simulink model "klademodel"  (R2023b)
settings: Solver=VariableStepAuto  StartTime=0.0  StopTime=50  RelTol=1e-3
libraries: simulink x1
settings Model: Creator=JesperBertelsen  LastModifiedBy=JesperBertelsen

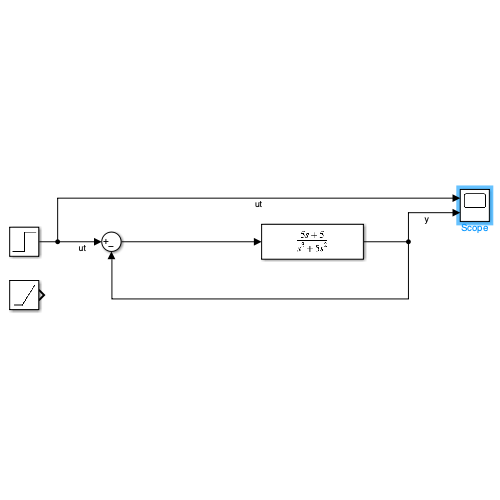
[thumbnail: Simulink's stored preview of the top-level diagram]
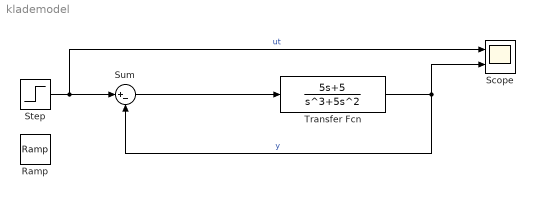
== system klademodel ==
  Ramp : simulink/Sources/Ramp  slope=10  start=0  InitialOutput=0
  Scope : Scope  NumInputPorts=2
  Step : Step  After=10  SampleTime=0
  Sum : Sum  Inputs=|+-
  Transfer Fcn : TransferFcn  Numerator=[5 5]  Denominator=[1 5 0 0]
  wires:
  Step/1 -> Scope/1, Sum/1  "ut"
  Transfer Fcn/1 -> Sum/2, Scope/2  "y"
  Sum/1 -> Transfer Fcn/1
